simulink model "INTEGRADOR_simu"  (R2021a)
settings: Solver=VariableStepAuto  StartTime=0.0  StopTime=100  MaxStep=1e-3  RelTol=1e-3
values from neighbouring files (symbols this model uses):
  G_den = [10 7 1]    [INTEGRADOR.m]    (also in matlab.mat)
  G_num = [1]    [INTEGRADOR.m]    (also in matlab.mat = 1)
  H_den = [1 2]    [INTEGRADOR.m]    (also in matlab.mat)
  H_num = [1]    [INTEGRADOR.m]    (also in matlab.mat = 1)
  tm_den = [1 1]    [matlab.mat]
  tm_num = [-1 1]    [matlab.mat]
settings Model: Creator=DELL  LastModifiedBy=DELL

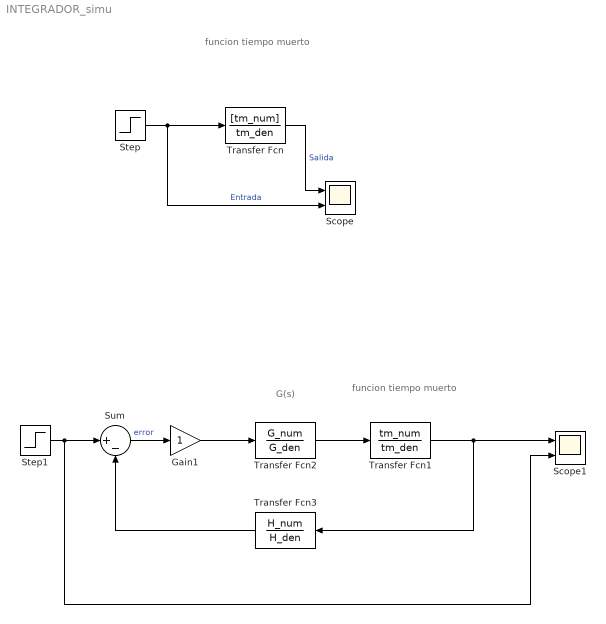
== system INTEGRADOR_simu ==
  note: G(s)
  note: funcion tiempo muerto
  note: funcion tiempo muerto
  Gain1 : Gain
  Scope : Scope  NumInputPorts=2
  Scope1 : Scope  NumInputPorts=2
  Step : Step  SampleTime=0
  Step1 : Step  SampleTime=0
  Sum : Sum  Inputs=|+-
  Transfer Fcn : TransferFcn  Numerator=[tm_num]  Denominator=tm_den
  Transfer Fcn1 : TransferFcn  Numerator=tm_num  Denominator=tm_den
  Transfer Fcn2 : TransferFcn  Numerator=G_num  Denominator=G_den
  Transfer Fcn3 : TransferFcn  Numerator=H_num  Denominator=H_den
  wires:
  Step/1 -> Scope/2, Transfer Fcn/1  "Entrada"
  Transfer Fcn/1 -> Scope/1  "Salida"
  Gain1/1 -> Transfer Fcn2/1
  Step1/1 -> Scope1/2, Sum/1
  Transfer Fcn1/1 -> Transfer Fcn3/1, Scope1/1
  Sum/1 -> Gain1/1  "error"
  Transfer Fcn2/1 -> Transfer Fcn1/1
  Transfer Fcn3/1 -> Sum/2
